simulink library "LevelDetectorLibraryLib"  (R2022b)
settings: Solver=VariableStepAuto  StartTime=0.0  StopTime=10.0  RelTol=1e-3
undefined symbols (not defined in the file or in its folder): Config
settings Model: Creator=bt1030690  LastModifiedBy=kl13806
settings SolverCC: AlgebraicLoopSolver=TrustRegion
settings DebuggingCC: UnconnectedInputMsg=warning  UnconnectedOutputMsg=warning  UnconnectedLineMsg=warning  SFMachineParentedDataDiag=warning  ArithmeticOperatorsInVariantConditions=warning
settings ModelReferenceCC: EnableRefExpFcnMdlSchedulingChecks=on
settings SFSimCC: SimUseLocalCustomCode=off  CustomCodeUndefinedFunction=UseInterfaceOnly
settings RTWCC: RTWUseLocalCustomCode=off  DLArmComputeVersion=19.05
settings CodeAppCC: StateflowObjectComments=on

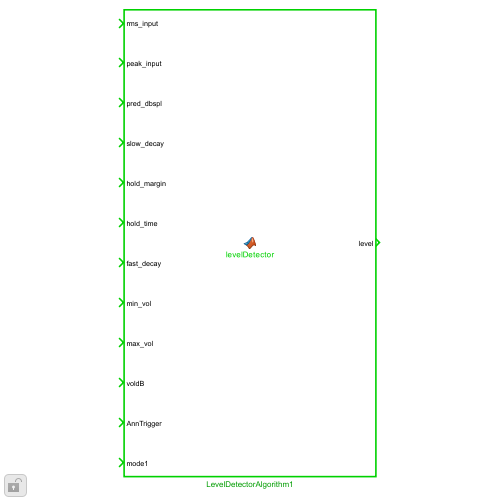
[thumbnail: Simulink's stored preview of the top-level diagram]
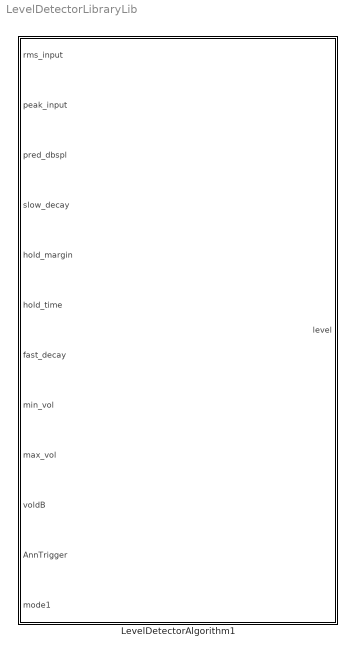
== system LevelDetectorLibraryLib ==
  LevelDetectorAlgorithm1 : MATLAB Function  TreatAsAtomicUnit=on  mask{Fd=Config.DlgDecRate}

== matlab function LevelDetectorLibraryLib/LevelDetectorAlgorithm1 ==
  data: rms_input input; peak_input input; pred_dbspl input; slow_decay input; hold_margin input; hold_time input; fast_decay input; min_vol input; max_vol input; voldB input; Fd parameter; AnnTrigger input; level output; mode1 input
function level  = levelDetector(rms_input, peak_input, pred_dbspl, ...
    slow_decay, hold_margin, hold_time, fast_decay, min_vol, max_vol, ...
    voldB, Fd, AnnTrigger, mode1)

% States
persistent holdFlag;
persistent holdState;
persistent env;

RMS_mode1 = single(1.0);
ANN_TRIGGER_THRESHOLD = single(0.5);

numberOfDetectors = 1;
SUPER_FAST_DECAY_MULTIPLIER =  single(3.0);

if (isempty(holdFlag))
    holdFlag = ones(numberOfDetectors,1);
    holdState = zeros(numberOfDetectors,1);
    env = -abs(min_vol)*ones(numberOfDetectors,1);
end

% Parameter conversion
%Fd = sys_defs.Fs / sys_defs.frameSize;

% Variable initialization
myMaxSPL = pred_dbspl;

mySlowDecay = single(zeros(numberOfDetectors,1));
myHoldMargin = single(zeros(numberOfDetectors,1));
myHoldTime = single(zeros(numberOfDetectors,1));
myFastDecay = single(zeros(numberOfDetectors,1));
myMinVol = single(zeros(numberOfDetectors,1));
myMaxVol = single(zeros(numberOfDetectors,1));
level = single(zeros(numberOfDetectors,1));
input1 = rms_input;

% Parameters for VNC level. 
mySlowDecay(1) = slow_decay;
myHoldMargin(1) = hold_margin;
myHoldTime(1) = hold_time;
myFastDecay(1) = fast_decay;
myMinVol(1) = min_vol;
myMaxVol(1) = max_vol;

%
% Slow Envelope - Fast attack, Hold with Very Slow Decay, Slow Decay
%

for k = 1:numberOfDetectors
   if mode1(k) > 0  
      if (mode1(k) > RMS_mode1)
         input1 = peak_input;
      end
   
      if (input1 >= (env(k) + myHoldMargin(k)))
         holdState(k) = 0;                  % reset state (but still decay)
      end
    
      if (input1 > env(k))
         env(k) = input1;                    % attack immediately
         holdFlag(k) = 1;                   % reset flag
         holdState(k) = 0;                  % reset state
      else
         holdState(k) = holdState(k) + 1;   % advance hold counter
         if ((holdState(k) > myHoldTime(k)) && ...
            ((env(k) + myHoldMargin(k)) > input1))
         holdFlag(k) = 0;                   %  end of hold
         end
         coef = mySlowDecay(k);             % slow decay
         if (holdFlag(k) == 0) || (AnnTrigger > ANN_TRIGGER_THRESHOLD)
            coef = myFastDecay(k);          % unless hold has ended OR Announcement trigger is ON
            if AnnTrigger > ANN_TRIGGER_THRESHOLD
               coef = SUPER_FAST_DECAY_MULTIPLIER*myFastDecay(k);
            end
         end    
         env(k) = env(k) + coef;            % compute new envelope      
      end    
      %
      % Bounds Check
      %    
      env(k) = max(myMinVol(k), env(k));
      env(k) = min(myMaxVol(k), env(k));
    
      %
      % dBSPL Conversion
      %    
      level(k) = max(0, env(k) + myMaxSPL + voldB);
   end    
end
